simulink model "tumblingExample"  (R2020a)
settings: Solver=ode8  StartTime=0.0  StopTime=1000  FixedStep=0.1  RelTol=1e-3
values from neighbouring files (symbols this model uses):
  a = sqrt(sum(aTimesOVec.^2))    [runDocking.m]
  b = params(3)    [a_max_CLVF3D.m]    (also in forGraphingSomeBasicStuff.m = 4; runDocking.m = 15)
  finalAngle = fact*pi    (= 2.98451302091)    [runDocking.m]
  J2 = -1.08264*10^-3    (= -0.00108264)    [runDocking.m]
  ka = params(1)    [a_max_CLVF3D.m]    (also in runDocking.m = 0.01)
  kc = params(2)    [a_max_CLVF3D.m]    (also in forGraphingSomeBasicStuff.m = 1; runDocking.m = 0.01)
  kd = 5.0    (= 5)    [runDocking.m]
  MU = 3.986 * 10^5    (= 398600)    [runDocking.m]
  o_hat_B = aTimesOVec./a    [runDocking.m]
  RC_I0 = rC_I0 + RT_I0    [runDocking.m]
  RE = 6378    [runDocking.m]
  v_max = interiorPointLVF_heur(a_prime, v_max, a_max, w_max, rotNorm, dockingPortNorm, theta_d, fact, W_LVF, mu, tol, gamma, beta, muFact, muLimit)    [runDocking.m]
  VC_I0 = vC_I0 + VT_I0    [runDocking.m]
undefined symbols (not defined in the file or in its folder): A_cone, A_d, a_max, a_prime, acceptableAngle, acceptableDistance, Aeq, beq_size, C_CB, CT_BI0, d, DiscIntNeverNeededParam, FixedStep, future_time_vector, J_transverse, J_z, K, LB, m, Np, o_hat_prime, Q, RT_I0, theta_d, u_con_mat, u_con_vec, UB, VT_I0, warm_start_matrix, wT_B0, X0, x_con_mat, x_con_vec
libraries: dspsigops x1, TBMPC_Blocks x1
settings Model: Creator=hough  LastModifiedBy=hough

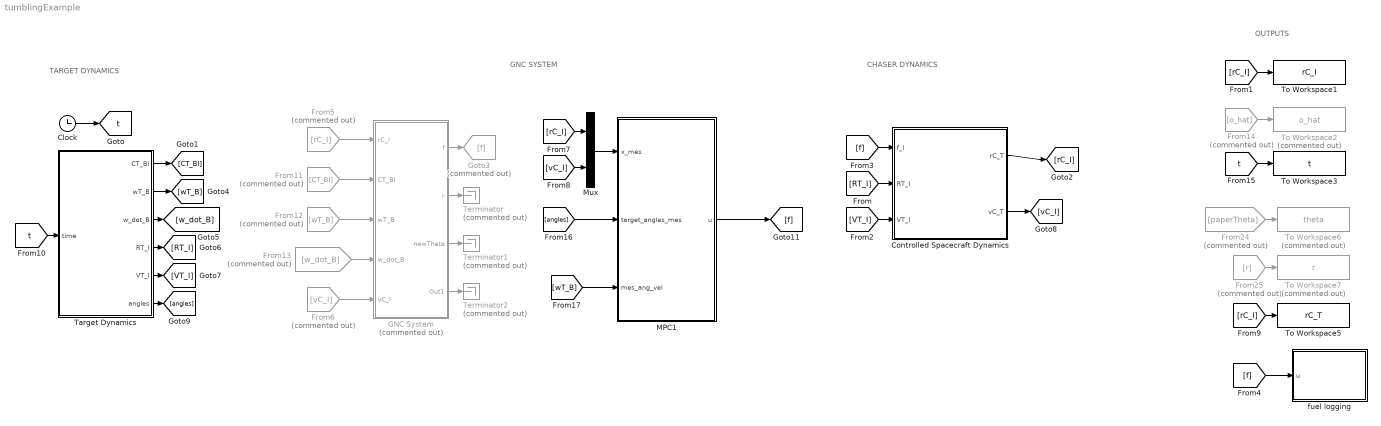
== system tumblingExample ==
  note: OUTPUTS
  note: GNC SYSTEM
  note: TARGET DYNAMICS
  note: CHASER DYNAMICS
  Clock : Clock
  Controlled Spacecraft Dynamics : Subsystem
  From11 : From  Commented=on  GotoTag=CT_BI
  From12 : From  Commented=on  GotoTag=wT_B
  From13 : From  Commented=on  GotoTag=w_dot_B
  From14 : From  Commented=on  GotoTag=o_hat
  From24 : From  Commented=on  GotoTag=paperTheta
  From25 : From  Commented=on  GotoTag=r
  From5 : From  Commented=on  GotoTag=rC_I
  From6 : From  Commented=on  GotoTag=vC_I
  GNC System : Subsystem  Commented=on
  Goto3 : Goto  Commented=on  GotoTag=f
  MPC1 : Subsystem  TreatAsAtomicUnit=on  SystemSampleTime=FixedStep  mask{t_vec=future_time_vector, J_z=J_z, J_transverse=J_transverse, u_con_mat=u_con_mat, u_con_vec=u_con_vec, x_con_mat_0=x_con_mat, x_con_vec=x_con_vec, Np=Np, d=d, A_cone=A_cone, Q=Q, Aeq=Aeq, warm_start_matrix=warm_start_matrix, A_discrete=A_d, K_feedback=K, X0=X0, beq_size=beq_size}
      mask prompts: t_vec "future time vector"; J_z "Inertia (sym axis)"; J_transverse "Inertia (trans axis)"; u_con_mat "u constraint matrix"; u_con_vec "u constraint vector"; x_con_mat_0 "x constraint matrix (proper size at least)"; x_con_vec "x constraint vector"; Np "Time horizon in steps"; d "Docking port in body-frame"; A_cone "Cone constraint matrix"; Q "Cost Matrix"; Aeq "Equality constraint matrix"; warm_start_matrix "warm start matrix"; A_discrete "A matrix (discrete system)"; K_feedback "Feedback Gain"; X0 "Initial optimizer guess"; beq_size "Height of equality matrix"
      mask help: This block runs a docking MPC controller for a axi-symmetric target spacecraft.
  Mux : Mux  Inputs=2
  Target Dynamics : Subsystem
  Terminator : Terminator  Commented=on
  Terminator1 : Terminator  Commented=on
  Terminator2 : Terminator  Commented=on
  To Workspace1 : ToWorkspace  VariableName=rC_I  SampleTime=-1
  To Workspace2 : ToWorkspace  Commented=on  VariableName=o_hat  SampleTime=-1
  To Workspace3 : ToWorkspace  VariableName=t  SampleTime=-1
  To Workspace5 : ToWorkspace  VariableName=rC_T  SampleTime=-1
  To Workspace6 : ToWorkspace  Commented=on  VariableName=theta  SampleTime=-1
  To Workspace7 : ToWorkspace  Commented=on  VariableName=r  SampleTime=-1
  fuel logging : Subsystem
  tag scope: t=global
  wires:
  GNC System/3(newTheta) -> Terminator1/1
  From12/1 -> GNC System/3(wT_B)
  From24/1 -> To Workspace6/1
  From13/1 -> GNC System/4(w_dot_B)
  From25/1 -> To Workspace7/1
  GNC System/2(r) -> Terminator/1
  [rC_I] -> To Workspace1/1
  From14/1 -> To Workspace2/1
  From11/1 -> GNC System/2(CT_BI)
  [t] -> To Workspace3/1
  Clock/1 -> [t]
  Target Dynamics/1(CT_BI) -> [CT_BI]
  Target Dynamics/2(wT_B) -> [wT_B]
  Target Dynamics/3(w_dot_B) -> [w_dot_B]
  [rC_I] -> To Workspace5/1
  Target Dynamics/4(RT_I) -> [RT_I]
  Target Dynamics/5(VT_I) -> [VT_I]
  [RT_I] -> Controlled Spacecraft Dynamics/2(RT_I)
  [VT_I] -> Controlled Spacecraft Dynamics/3(VT_I)
  GNC System/1(f) -> Goto3/1
  [f] -> Controlled Spacecraft Dynamics/1(f_I)
  [f] -> fuel logging/1(u)
  From5/1 -> GNC System/1(rC_I)
  Controlled Spacecraft Dynamics/2(vC_T) -> [vC_I]
  From6/1 -> GNC System/5(vC_I)
  [rC_I] -> Mux/1
  [vC_I] -> Mux/2
  Mux/1 -> MPC1/1(x_mes)
  GNC System/4(Out1) -> Terminator2/1
  [t] -> Target Dynamics/1(time)
  Target Dynamics/6(angles) -> [angles]
  [angles] -> MPC1/2(target_angles_mes)
  [wT_B] -> MPC1/3(mes_ang_vel)
  MPC1/1(u) -> [f]
  Controlled Spacecraft Dynamics/1(rC_T) -> [rC_I]

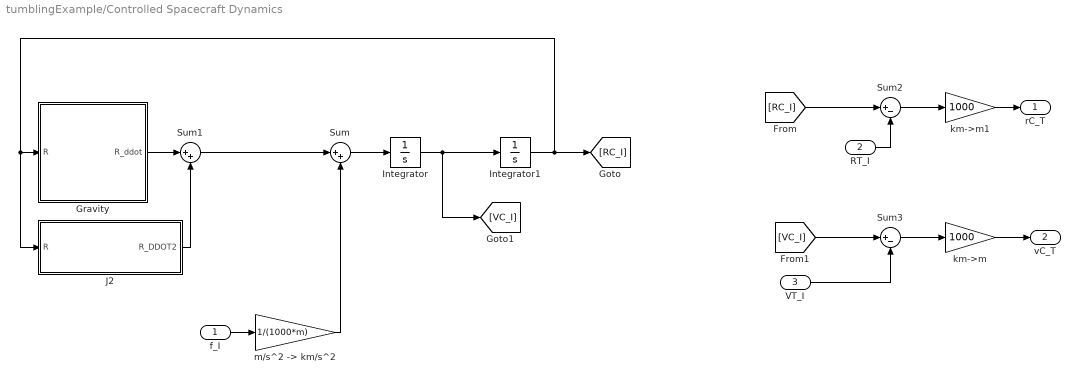
== system tumblingExample/Controlled Spacecraft Dynamics ==
  f_I : Inport
  RT_I : Inport  Port=2
  VT_I : Inport  Port=3
  Gravity : MATLAB Function  TreatAsAtomicUnit=on
  Integrator : Integrator  InitialCondition=VC_I0
  Integrator1 : Integrator  InitialCondition=RC_I0
  J2 : MATLAB Function  TreatAsAtomicUnit=on
  Sum : Sum  Inputs=|++
  Sum1 : Sum  Inputs=|++
  Sum2 : Sum  Inputs=|+-
  Sum3 : Sum  Inputs=|+-
  km->m : Gain  Gain=1000
  km->m1 : Gain  Gain=1000
  "m/s^2 -> km/s^2" : Gain  Gain=1/(1000*m)
  rC_T : Outport
  vC_T : Outport  Port=2
  wires:
  Integrator1/1 -> Gravity/1(R), J2/1(R), [RC_I]
  Integrator/1 -> Integrator1/1, [VC_I]
  Sum/1 -> Integrator/1
  f_I/1 -> "m/s^2 -> km/s^2"/1
  Gravity/1(R_ddot) -> Sum1/1
  J2/1(R_DDOT2) -> Sum1/2
  "m/s^2 -> km/s^2"/1 -> Sum/2
  Sum2/1 -> km->m1/1
  RT_I/1 -> Sum2/2
  [RC_I] -> Sum2/1
  km->m1/1 -> rC_T/1
  Sum3/1 -> km->m/1
  VT_I/1 -> Sum3/2
  [VC_I] -> Sum3/1
  km->m/1 -> vC_T/1
  Sum1/1 -> Sum/1

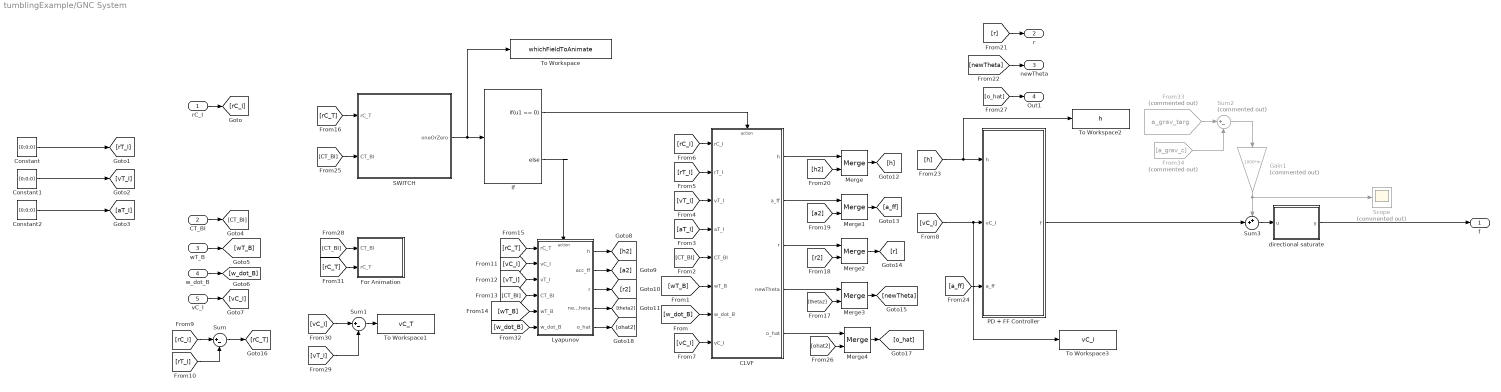
== system tumblingExample/GNC System ==
  rC_I : Inport
  CT_BI : Inport  Port=2
  wT_B : Inport  Port=3
  w_dot_B : Inport  Port=4
  vC_I : Inport  Port=5
  CLVF : Subsystem
  Constant : Constant  Value=[0;0;0]
  Constant1 : Constant  Value=[0;0;0]
  Constant2 : Constant  Value=[0;0;0]
  For Animation : Subsystem
  From33 : From  Commented=on  GotoTag=a_grav_targ  TagVisibility=global
  From34 : From  Commented=on  GotoTag=a_grav_c  TagVisibility=global
  Gain1 : Gain  Commented=on  Gain=1000*m
  If : If  IfExpression=u1 == 0
  Lyapunov : Subsystem  TreatAsAtomicUnit=on
  Merge{,1..4} (5 alike) : Merge
  PD + FF Controller : MATLAB Function  TreatAsAtomicUnit=on
  SWITCH : Subsystem
  Scope : Scope  Commented=on
  Sum : Sum  Inputs=|+-
  Sum1 : Sum  Inputs=|+-
  Sum2 : Sum  Commented=on  Inputs=|+-
  Sum3 : Sum  Inputs=++|
  To Workspace : ToWorkspace  VariableName=whichFieldToAnimate  SampleTime=-1
  To Workspace1 : ToWorkspace  VariableName=vC_T  SampleTime=-1
  To Workspace2 : ToWorkspace  VariableName=h  SampleTime=-1
  To Workspace3 : ToWorkspace  VariableName=vC_I  SampleTime=-1
  directional saturate : MATLAB Function  TreatAsAtomicUnit=on
  f : Outport
  r : Outport  Port=2
  newTheta : Outport  Port=3
  Out1 : Outport  Port=4
  wires:
  rC_I/1 -> [rC_I]
  CT_BI/1 -> [CT_BI]
  wT_B/1 -> [wT_B]
  w_dot_B/1 -> [w_dot_B]
  vC_I/1 -> [vC_I]
  [vC_I] -> To Workspace3/1, PD + FF Controller/2(vC_I)
  [rC_I] -> CLVF/1(rC_I)
  [rT_I] -> CLVF/2(rT_I)
  [vT_I] -> CLVF/3(vT_I)
  [aT_I] -> CLVF/4(aT_I)
  [CT_BI] -> CLVF/5(CT_BI)
  [wT_B] -> CLVF/6(wT_B)
  [w_dot_B] -> CLVF/7(w_dot_B)
  [vC_I] -> CLVF/8(vC_I)
  If/1 -> CLVF/Action
  CLVF/1(h) -> Merge/1
  CLVF/2(a_ff) -> Merge1/1
  CLVF/3(r) -> Merge2/1
  CLVF/4(newTheta) -> Merge3/1
  [theta2] -> Merge3/2
  [r2] -> Merge2/2
  [a2] -> Merge1/2
  [h2] -> Merge/2
  Merge/1 -> [h]
  Merge1/1 -> [a_ff]
  Merge2/1 -> [r]
  Merge3/1 -> [newTheta]
  [r] -> r/1
  [newTheta] -> newTheta/1
  [h] -> To Workspace2/1, PD + FF Controller/1(h)
  [a_ff] -> PD + FF Controller/3(a_ff)
  If/2 -> Lyapunov/Action
  [rC_I] -> Sum/1
  [rT_I] -> Sum/2
  Lyapunov/1(h) -> [h2]
  Lyapunov/2(acc_ff) -> [a2]
  Lyapunov/3(r) -> [r2]
  Lyapunov/4(newTheta) -> [theta2]
  [vC_I] -> Lyapunov/2(vC_I)
  [vT_I] -> Lyapunov/3(vT_I)
  SWITCH/1(oneOrZero) -> To Workspace/1, If/1
  Sum/1 -> [rC_T]
  [rC_T] -> Lyapunov/1(rC_T)
  [rC_T] -> SWITCH/1(rC_T)
  Merge4/1 -> [o_hat]
  CLVF/5(o_hat) -> Merge4/1
  [ohat2] -> Merge4/2
  Lyapunov/5(o_hat) -> [ohat2]
  [o_hat] -> Out1/1
  [vC_I] -> Sum1/1
  [vT_I] -> Sum1/2
  Sum1/1 -> To Workspace1/1
  [rC_T] -> For Animation/2(rC_T)
  [CT_BI] -> Lyapunov/4(CT_BI)
  [wT_B] -> Lyapunov/5(wT_B)
  [w_dot_B] -> Lyapunov/6(w_dot_B)
  [CT_BI] -> SWITCH/2(CT_BI)
  [CT_BI] -> For Animation/1(CT_BI)
  PD + FF Controller/1(f) -> Sum3/2
  directional saturate/1(y) -> f/1
  Sum2/1 -> Gain1/1
  From34/1 -> Sum2/2
  From33/1 -> Sum2/1
  Gain1/1 -> Sum3/1, Scope/1
  Sum3/1 -> directional saturate/1(u)
  Constant/1 -> [rT_I]
  Constant1/1 -> [vT_I]
  Constant2/1 -> [aT_I]

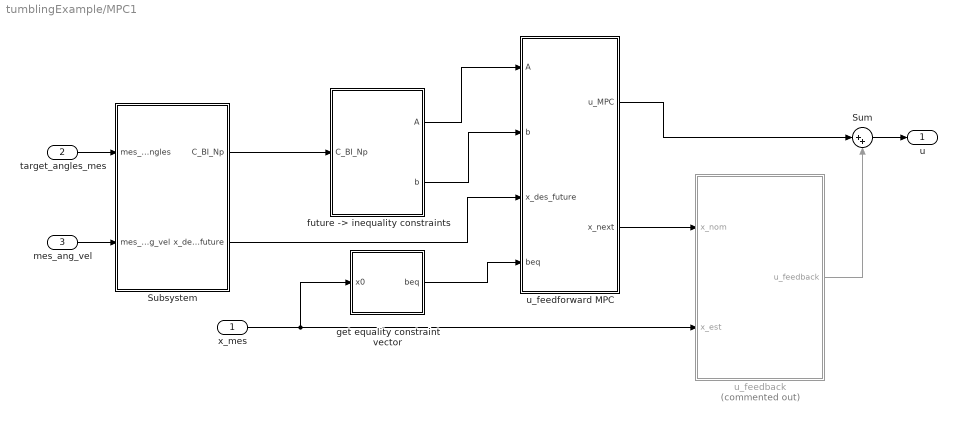
== system tumblingExample/MPC1 ==
  x_mes : Inport
  target_angles_mes : Inport  Port=2
  mes_ang_vel : Inport  Port=3
  Subsystem : Subsystem
  Sum : Sum  Inputs=|++
  "future -> inequality constraints" : Subsystem
  get equality constraint vector : Subsystem
  u_feedback : Subsystem  Commented=on
  u_feedforward MPC : Subsystem
  u : Outport
  wires:
  u_feedforward MPC/1(u_MPC) -> Sum/1
  Sum/1 -> u/1
  x_mes/1 -> get equality constraint vector/1(x0), u_feedback/2(x_est)
  u_feedforward MPC/2(x_next) -> u_feedback/1(x_nom)
  u_feedback/1(u_feedback) -> Sum/2
  "future -> inequality constraints"/1(A) -> u_feedforward MPC/1(A)
  "future -> inequality constraints"/2(b) -> u_feedforward MPC/2(b)
  Subsystem/1(C_BI_Np) -> "future -> inequality constraints"/1(C_BI_Np)
  target_angles_mes/1 -> Subsystem/1(mes_angles)
  mes_ang_vel/1 -> Subsystem/2(mes_ang_vel)
  Subsystem/2(x_des_future) -> u_feedforward MPC/3(x_des_future)
  get equality constraint vector/1(beq) -> u_feedforward MPC/4(beq)

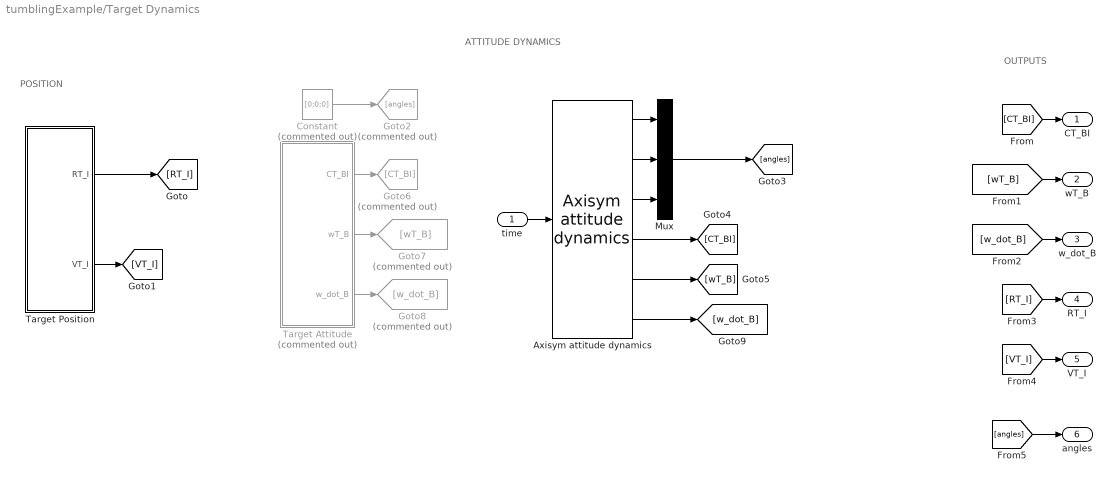
== system tumblingExample/Target Dynamics ==
  note: POSITION
  note: ATTITUDE DYNAMICS
  note: OUTPUTS
  time : Inport
  Axisym attitude dynamics : TBMPC_Blocks/Axisym attitude dynamics  J_transverse=J_transverse  J_z=J_z  omega_t=w_t  omega_z=w_z  mu_0=mu0  gamma_0=gamma  theta_0=theta0
  Constant : Constant  Commented=on  Value=[0;0;0]
  Goto2 : Goto  Commented=on  GotoTag=angles
  Goto6 : Goto  Commented=on  GotoTag=CT_BI
  Goto7 : Goto  Commented=on  GotoTag=wT_B
  Goto8 : Goto  Commented=on  GotoTag=w_dot_B
  Mux : Mux  Inputs=3
  Target Attitude : Subsystem  Commented=on
  Target Position : Subsystem
  CT_BI : Outport
  wT_B : Outport  Port=2
  w_dot_B : Outport  Port=3
  RT_I : Outport  Port=4
  VT_I : Outport  Port=5
  angles : Outport  Port=6
  wires:
  Target Attitude/3(w_dot_B) -> Goto8/1
  Target Attitude/1(CT_BI) -> Goto6/1
  Target Attitude/2(wT_B) -> Goto7/1
  [CT_BI] -> CT_BI/1
  [wT_B] -> wT_B/1
  [w_dot_B] -> w_dot_B/1
  Target Position/2(VT_I) -> [VT_I]
  [RT_I] -> RT_I/1
  [VT_I] -> VT_I/1
  time/1 -> Axisym attitude dynamics/1
  Axisym attitude dynamics/1 -> Mux/1
  Axisym attitude dynamics/2 -> Mux/2
  Axisym attitude dynamics/3 -> Mux/3
  [angles] -> angles/1
  Constant/1 -> Goto2/1
  Mux/1 -> [angles]
  Axisym attitude dynamics/4 -> [CT_BI]
  Axisym attitude dynamics/5 -> [wT_B]
  Axisym attitude dynamics/6 -> [w_dot_B]
  Target Position/1(RT_I) -> [RT_I]

== system tumblingExample/fuel logging ==
  u : Inport
  F->acc : Gain  Gain=1/m
  Gain : Gain  Gain=1/m
  To Workspace4 : ToWorkspace  VariableName=a_norm  SampleTime=-1
  To Workspace8 : ToWorkspace  VariableName=F_act  SampleTime=-1
  acc->delV : DiscreteIntegrator  SampleTime=-1  ICPrevOutput=DiscIntNeverNeededParam  ICPrevScaledInput=DiscIntNeverNeededParam
  get Norm : MATLAB Function  TreatAsAtomicUnit=on
  getNorm : MATLAB Function  TreatAsAtomicUnit=on
  wires:
  getNorm/1(y) -> Gain/1
  get Norm/1(y) -> acc->delV/1
  acc->delV/1 -> To Workspace8/1
  F->acc/1 -> get Norm/1(u)
  Gain/1 -> To Workspace4/1
  u/1 -> F->acc/1, getNorm/1(u)

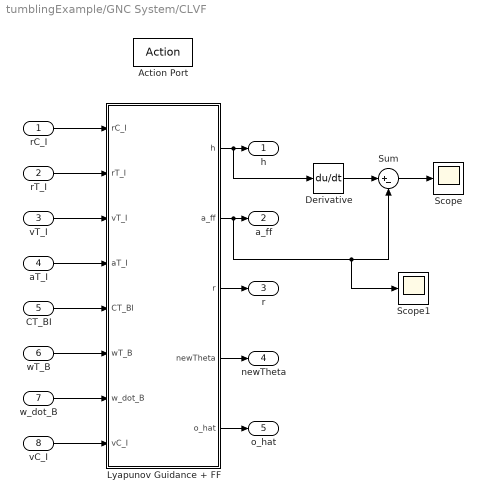
== system tumblingExample/GNC System/CLVF ==
  rC_I : Inport
  rT_I : Inport  Port=2
  vT_I : Inport  Port=3
  aT_I : Inport  Port=4
  CT_BI : Inport  Port=5
  wT_B : Inport  Port=6
  w_dot_B : Inport  Port=7
  vC_I : Inport  Port=8
  Action Port : ActionPort  ActionPortLabel=if(u1 == 0)
  Derivative : Derivative
  Lyapunov Guidance + FF : MATLAB Function  TreatAsAtomicUnit=on
  Scope : Scope
  Scope1 : Scope
  Sum : Sum  Inputs=|+-
  h : Outport
  a_ff : Outport  Port=2
  r : Outport  Port=3
  newTheta : Outport  Port=4
  o_hat : Outport  Port=5
  wires:
  vT_I/1 -> Lyapunov Guidance + FF/3(vT_I)
  rT_I/1 -> Lyapunov Guidance + FF/2(rT_I)
  wT_B/1 -> Lyapunov Guidance + FF/6(wT_B)
  w_dot_B/1 -> Lyapunov Guidance + FF/7(w_dot_B)
  vC_I/1 -> Lyapunov Guidance + FF/8(vC_I)
  CT_BI/1 -> Lyapunov Guidance + FF/5(CT_BI)
  aT_I/1 -> Lyapunov Guidance + FF/4(aT_I)
  rC_I/1 -> Lyapunov Guidance + FF/1(rC_I)
  Lyapunov Guidance + FF/3(r) -> r/1
  Lyapunov Guidance + FF/2(a_ff) -> Scope1/1, Sum/2, a_ff/1
  Lyapunov Guidance + FF/1(h) -> Derivative/1, h/1
  Lyapunov Guidance + FF/4(newTheta) -> newTheta/1
  Lyapunov Guidance + FF/5(o_hat) -> o_hat/1
  Derivative/1 -> Sum/1
  Sum/1 -> Scope/1

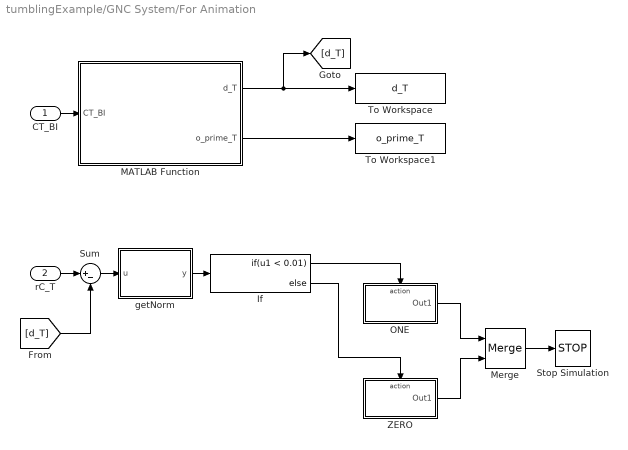
== system tumblingExample/GNC System/For Animation ==
  CT_BI : Inport
  rC_T : Inport  Port=2
  If : If  IfExpression=u1 < 0.01
  MATLAB Function : MATLAB Function  TreatAsAtomicUnit=on
  Merge : Merge
  ONE : Subsystem  TreatAsAtomicUnit=on
  Stop Simulation : Stop
  Sum : Sum  Inputs=|+-
  To Workspace : ToWorkspace  VariableName=d_T  SampleTime=-1
  To Workspace1 : ToWorkspace  VariableName=o_prime_T  SampleTime=-1
  ZERO : Subsystem  TreatAsAtomicUnit=on
  getNorm : MATLAB Function  TreatAsAtomicUnit=on
  wires:
  CT_BI/1 -> MATLAB Function/1(CT_BI)
  MATLAB Function/1(d_T) -> [d_T], To Workspace/1
  MATLAB Function/2(o_prime_T) -> To Workspace1/1
  rC_T/1 -> Sum/1
  [d_T] -> Sum/2
  Sum/1 -> getNorm/1(u)
  getNorm/1(y) -> If/1
  If/1 -> ONE/Action
  If/2 -> ZERO/Action
  ONE/1(Out1) -> Merge/1
  ZERO/1(Out1) -> Merge/2
  Merge/1 -> Stop Simulation/1

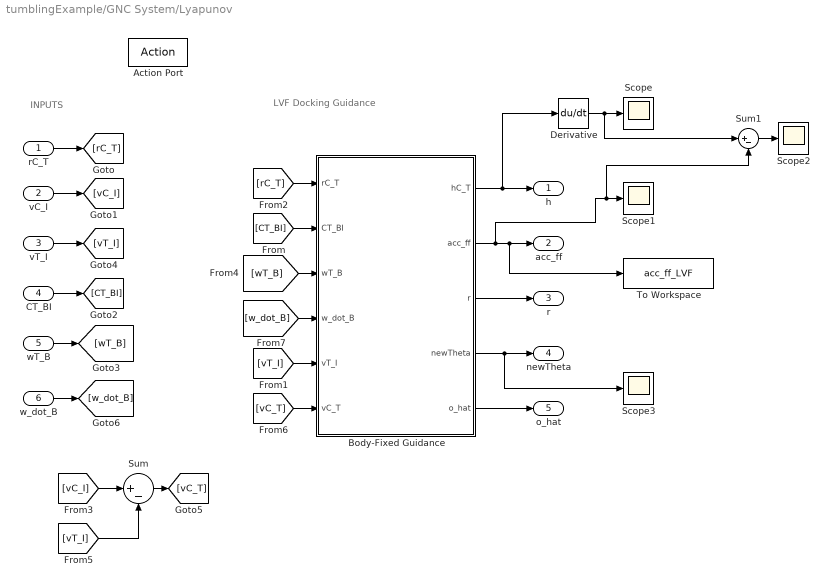
== system tumblingExample/GNC System/Lyapunov ==
  note: LVF Docking Guidance
  note: INPUTS
  rC_T : Inport
  vC_I : Inport  Port=2
  vT_I : Inport  Port=3
  CT_BI : Inport  Port=4
  wT_B : Inport  Port=5
  w_dot_B : Inport  Port=6
  Action Port : ActionPort  ActionPortLabel=else
  Body-Fixed Guidance : MATLAB Function  TreatAsAtomicUnit=on
  Derivative : Derivative
  Scope{,1..3} (4 alike) : Scope
  Sum : Sum  Inputs=|+-
  Sum1 : Sum  Inputs=|+-
  To Workspace : ToWorkspace  VariableName=acc_ff_LVF  SampleTime=-1
  h : Outport
  acc_ff : Outport  Port=2
  r : Outport  Port=3
  newTheta : Outport  Port=4
  o_hat : Outport  Port=5
  wires:
  rC_T/1 -> [rC_T]
  vC_I/1 -> [vC_I]
  CT_BI/1 -> [CT_BI]
  wT_B/1 -> [wT_B]
  [rC_T] -> Body-Fixed Guidance/1(rC_T)
  [wT_B] -> Body-Fixed Guidance/3(wT_B)
  [CT_BI] -> Body-Fixed Guidance/2(CT_BI)
  [w_dot_B] -> Body-Fixed Guidance/4(w_dot_B)
  vT_I/1 -> [vT_I]
  Body-Fixed Guidance/1(hC_T) -> Derivative/1, h/1
  [vT_I] -> Body-Fixed Guidance/5(vT_I)
  Body-Fixed Guidance/3(r) -> r/1
  Body-Fixed Guidance/4(newTheta) -> Scope3/1, newTheta/1
  Body-Fixed Guidance/5(o_hat) -> o_hat/1
  [vC_I] -> Sum/1
  [vT_I] -> Sum/2
  Sum/1 -> [vC_T]
  [vC_T] -> Body-Fixed Guidance/6(vC_T)
  Body-Fixed Guidance/2(acc_ff) -> To Workspace/1, acc_ff/1, Sum1/2, Scope1/1
  Derivative/1 -> Sum1/1, Scope/1
  Sum1/1 -> Scope2/1
  w_dot_B/1 -> [w_dot_B]

== system tumblingExample/GNC System/SWITCH ==
  rC_T : Inport
  CT_BI : Inport  Port=2
  Delay : Delay  DelayLength=1  InitialCondition=0
  Sample and Hold : dspsigops/Sample and Hold  trig=Rising edge  initCond=0  latchinput=off
  inDesiredRadius : MATLAB Function  TreatAsAtomicUnit=on
  sufficientTime : MATLAB Function  TreatAsAtomicUnit=on
  oneOrZero : Outport
  wires:
  rC_T/1 -> inDesiredRadius/1(rC_T)
  CT_BI/1 -> inDesiredRadius/2(CT_BI)
  Delay/1 -> inDesiredRadius/3(currentCnt)
  inDesiredRadius/1(newCnt) -> sufficientTime/1(cnt), Delay/1
  Sample and Hold/1 -> oneOrZero/1
  sufficientTime/1(oneOrZero) -> Sample and Hold/Trigger, Sample and Hold/1

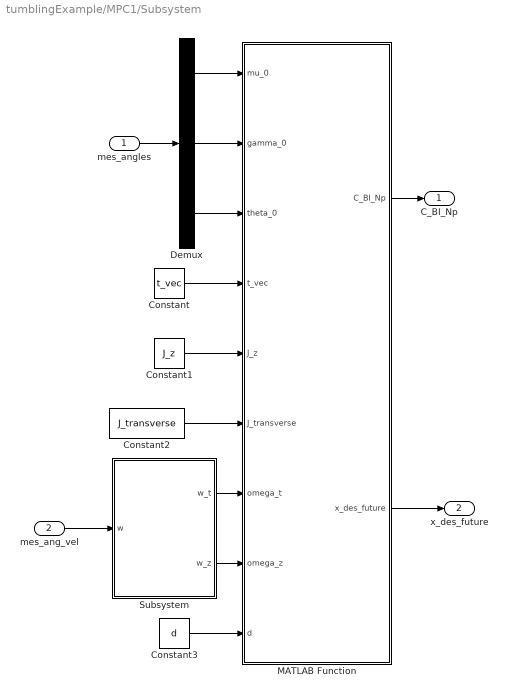
== system tumblingExample/MPC1/Subsystem ==
  mes_angles : Inport
  mes_ang_vel : Inport  Port=2
  Constant : Constant  Value=t_vec
  Constant1 : Constant  Value=J_z
  Constant2 : Constant  Value=J_transverse
  Constant3 : Constant  Value=d
  Demux : Demux  Outputs=3
  MATLAB Function : MATLAB Function  TreatAsAtomicUnit=on
  Subsystem : Subsystem
  C_BI_Np : Outport
  x_des_future : Outport  Port=2
  wires:
  MATLAB Function/1(C_BI_Np) -> C_BI_Np/1
  MATLAB Function/2(x_des_future) -> x_des_future/1
  Constant/1 -> MATLAB Function/4(t_vec)
  Demux/2 -> MATLAB Function/2(gamma_0)
  Demux/3 -> MATLAB Function/3(theta_0)
  Demux/1 -> MATLAB Function/1(mu_0)
  mes_angles/1 -> Demux/1
  Constant2/1 -> MATLAB Function/6(J_transverse)
  Constant1/1 -> MATLAB Function/5(J_z)
  mes_ang_vel/1 -> Subsystem/1(w)
  Subsystem/1(w_t) -> MATLAB Function/7(omega_t)
  Subsystem/2(w_z) -> MATLAB Function/8(omega_z)
  Constant3/1 -> MATLAB Function/9(d)

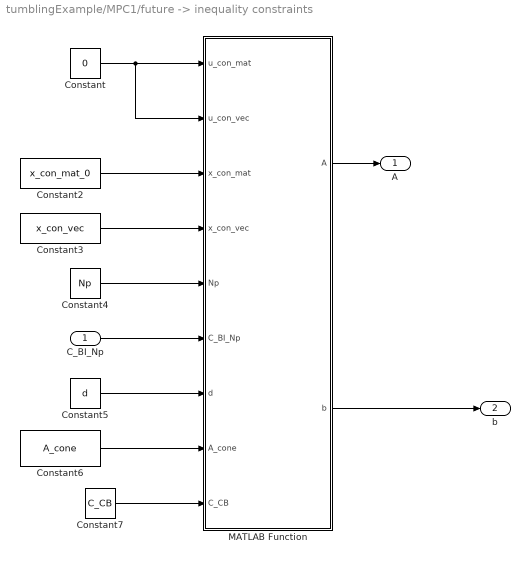
== system tumblingExample/MPC1/future -> inequality constraints ==
  C_BI_Np : Inport
  Constant : Constant  Value=0
  Constant2 : Constant  Value=x_con_mat_0
  Constant3 : Constant  Value=x_con_vec
  Constant4 : Constant  Value=Np
  Constant5 : Constant  Value=d
  Constant6 : Constant  Value=A_cone
  Constant7 : Constant  Value=C_CB
  MATLAB Function : MATLAB Function  TreatAsAtomicUnit=on
  A : Outport
  b : Outport  Port=2
  wires:
  MATLAB Function/1(A) -> A/1
  C_BI_Np/1 -> MATLAB Function/6(C_BI_Np)
  Constant2/1 -> MATLAB Function/3(x_con_mat)
  Constant3/1 -> MATLAB Function/4(x_con_vec)
  Constant4/1 -> MATLAB Function/5(Np)
  Constant5/1 -> MATLAB Function/7(d)
  Constant6/1 -> MATLAB Function/8(A_cone)
  Constant7/1 -> MATLAB Function/9(C_CB)
  MATLAB Function/2(b) -> b/1
  Constant/1 -> MATLAB Function/2(u_con_vec), MATLAB Function/1(u_con_mat)

== system tumblingExample/MPC1/get equality constraint vector ==
  x0 : Inport
  Constant : Constant  Value=Np
  Constant1 : Constant  Value=A_discrete
  Gain : Gain  Gain=-1
  MATLAB Function : MATLAB Function  TreatAsAtomicUnit=on
  beq : Outport
  wires:
  x0/1 -> MATLAB Function/3(x0)
  Constant/1 -> MATLAB Function/2(Np)
  Constant1/1 -> MATLAB Function/1(A)
  Gain/1 -> beq/1
  MATLAB Function/1(p) -> Gain/1

== system tumblingExample/MPC1/u_feedback ==
  x_nom : Inport
  x_est : Inport  Port=2
  Constant : Constant  Value=K_feedback
  Matrix Multiply : Product  Multiplication=Matrix(*)
  Sum : Sum  Inputs=|+-
  u_feedback : Outport
  wires:
  x_nom/1 -> Sum/1
  x_est/1 -> Sum/2
  Sum/1 -> Matrix Multiply/2
  Constant/1 -> Matrix Multiply/1
  Matrix Multiply/1 -> u_feedback/1

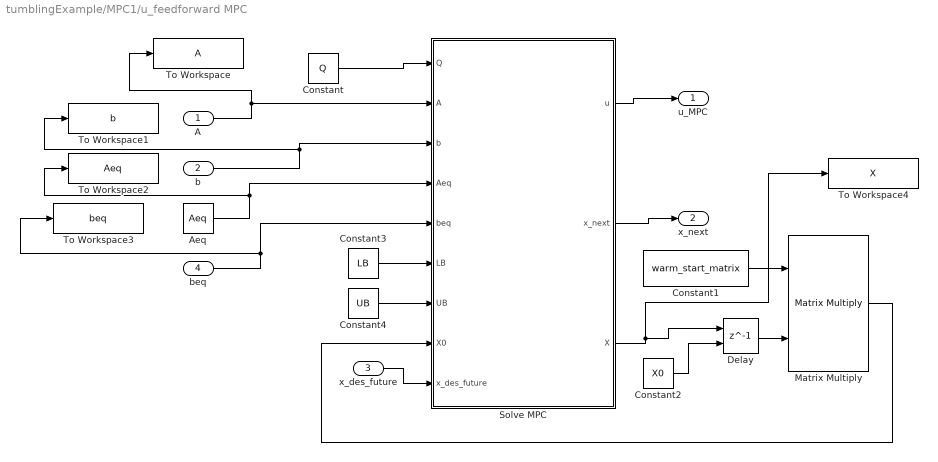
== system tumblingExample/MPC1/u_feedforward MPC ==
  A : Inport
  b : Inport  Port=2
  x_des_future : Inport  Port=3
  beq : Inport  Port=4
  Aeq : Constant  Value=Aeq
  Constant : Constant  Value=Q
  Constant1 : Constant  Value=warm_start_matrix
  Constant2 : Constant  Value=X0
  Constant3 : Constant  Value=LB
  Constant4 : Constant  Value=UB
  Delay : Delay  DelayLength=1  InitialConditionSource=Input port
      settings: InputPortMap=u0,p4
  Matrix Multiply : Product  Multiplication=Matrix(*)
  Solve MPC : MATLAB Function  TreatAsAtomicUnit=on
  To Workspace : ToWorkspace  VariableName=A  SaveFormat=Structure  SampleTime=-1
  To Workspace1 : ToWorkspace  VariableName=b  SaveFormat=Structure  SampleTime=-1
  To Workspace2 : ToWorkspace  VariableName=Aeq  SampleTime=-1
  To Workspace3 : ToWorkspace  VariableName=beq  SaveFormat=Structure  SampleTime=-1
  To Workspace4 : ToWorkspace  VariableName=X  SampleTime=-1
  u_MPC : Outport
  x_next : Outport  Port=2
  wires:
  A/1 -> To Workspace/1, Solve MPC/2(A)
  Matrix Multiply/1 -> Solve MPC/8(X0)
  beq/1 -> To Workspace3/1, Solve MPC/5(beq)
  Constant1/1 -> Matrix Multiply/1
  Constant/1 -> Solve MPC/1(Q)
  Delay/1 -> Matrix Multiply/2
  Aeq/1 -> To Workspace2/1, Solve MPC/4(Aeq)
  b/1 -> To Workspace1/1, Solve MPC/3(b)
  Solve MPC/3(X) -> To Workspace4/1, Delay/1
  Solve MPC/1(u) -> u_MPC/1
  Solve MPC/2(x_next) -> x_next/1
  x_des_future/1 -> Solve MPC/9(x_des_future)
  Constant2/1 -> Delay/2
  Constant3/1 -> Solve MPC/6(LB)
  Constant4/1 -> Solve MPC/7(UB)

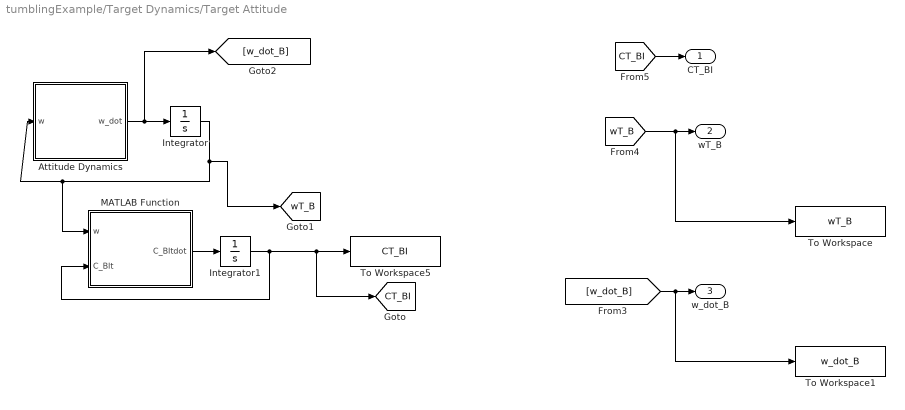
== system tumblingExample/Target Dynamics/Target Attitude ==
  Attitude Dynamics : MATLAB Function  TreatAsAtomicUnit=on
  Integrator : Integrator  InitialCondition=wT_B0
  Integrator1 : Integrator  InitialCondition=CT_BI0
  MATLAB Function : MATLAB Function  TreatAsAtomicUnit=on
  To Workspace : ToWorkspace  VariableName=wT_B  SampleTime=-1
  To Workspace1 : ToWorkspace  VariableName=w_dot_B  SampleTime=-1
  To Workspace5 : ToWorkspace  VariableName=CT_BI  SampleTime=-1
  CT_BI : Outport
  wT_B : Outport  Port=2
  w_dot_B : Outport  Port=3
  tag scope: CT_BI=global, wT_B=global
  wires:
  [CT_BI] -> CT_BI/1
  [wT_B] -> To Workspace/1, wT_B/1
  [w_dot_B] -> To Workspace1/1, w_dot_B/1
  MATLAB Function/1(C_BItdot) -> Integrator1/1
  Integrator1/1 -> MATLAB Function/2(C_BIt), [CT_BI], To Workspace5/1
  Integrator/1 -> [wT_B], MATLAB Function/1(w), Attitude Dynamics/1(w)
  Attitude Dynamics/1(w_dot) -> [w_dot_B], Integrator/1

== system tumblingExample/Target Dynamics/Target Position ==
  Gravity : MATLAB Function  TreatAsAtomicUnit=on
  Integrator : Integrator  InitialCondition=VT_I0
  Integrator1 : Integrator  InitialCondition=RT_I0
  J2 : MATLAB Function  TreatAsAtomicUnit=on
  Sum : Sum  Inputs=|++
  RT_I : Outport
  VT_I : Outport  Port=2
  tag scope: a_grav_targ=global
  wires:
  Integrator/1 -> VT_I/1, Integrator1/1
  Integrator1/1 -> RT_I/1, J2/1(R), Gravity/1(R)
  Gravity/1(R_ddot) -> Sum/1
  J2/1(R_DDOT2) -> Sum/2
  Sum/1 -> [a_grav_targ], Integrator/1

== system tumblingExample/GNC System/For Animation/ONE ==
  Action Port : ActionPort  ActionPortLabel=if(u1 < 0.01)
  Constant : Constant
  Out1 : Outport
  wires:
  Constant/1 -> Out1/1

== system tumblingExample/GNC System/For Animation/ZERO ==
  Action Port : ActionPort  ActionPortLabel=else
  Constant : Constant  Value=0
  Out1 : Outport
  wires:
  Constant/1 -> Out1/1

== system tumblingExample/MPC1/Subsystem/Subsystem ==
  w : Inport
  Add : Sum
  Demux1 : Demux  Outputs=3
  Sqrt : Sqrt  SaturateOnIntegerOverflow=on
  Square : Math  Operator=square  SaturateOnIntegerOverflow=on
  Square1 : Math  Operator=square  SaturateOnIntegerOverflow=on
  w_t : Outport
  w_z : Outport  Port=2
  wires:
  Square/1 -> Add/1
  Demux1/1 -> Square/1
  Demux1/2 -> Square1/1
  Add/1 -> Sqrt/1
  Square1/1 -> Add/2
  w/1 -> Demux1/1
  Demux1/3 -> w_z/1
  Sqrt/1 -> w_t/1

== matlab function tumblingExample/MPC1/Subsystem/MATLAB Function ==
  data: mu_0 input; C_BI_Np output; gamma_0 input; theta_0 input; t_vec input; J_z input; J_transverse input; omega_t input; omega_z input; x_des_future output; d input
function [C_BI_Np, x_des_future] = fcn(mu_0, gamma_0, theta_0, t_vec, J_z, J_transverse, omega_t, omega_z, d)

    [C_BI_Np, x_des_future] = return_C_BI_from_axisym(mu_0, gamma_0, theta_0, t_vec, J_z, J_transverse, omega_z, omega_t, d);


end

== matlab function tumblingExample/Target Dynamics/Target Attitude/MATLAB Function ==
  data: w input; C_BItdot output; C_BIt input
function C_BItdot = fcn(w,C_BIt)

w_skew = [0 -w(3) w(2)
          w(3) 0 -w(1)
          -w(2) w(1) 0];

C_BItdot = -w_skew*C_BIt;

== matlab function tumblingExample/GNC System/SWITCH/sufficientTime ==
  data: oneOrZero output; cnt input; cntThreshold parameter
function oneOrZero = fcn(cnt, cntThreshold)

    if cnt < cntThreshold
        oneOrZero = 0; % Not enough.
    else
        oneOrZero = 1;
    end
end

== matlab function tumblingExample/fuel logging/getNorm ==
  data: u input; y output
function y = fcn(u)

y = sqrt(sum(u.^2));

== matlab function tumblingExample/Controlled Spacecraft Dynamics/J2 ==
  data: R input; R_DDOT2 output; MU parameter; J2 parameter; RE parameter
function R_DDOT2 = fcn(R, MU, J2, RE)

R_norm = sqrt(sum(R.^2));

R_DDOT2_part1 = 3*MU*J2*RE^2/(2*R_norm^5);

R_DDOT2_part2 = (  5*(R(3))^2/R_norm^2  -  1  )*R;

R_DDOT2_part3 =  -2*R(3)*[0;0;1];

R_DDOT2 = R_DDOT2_part1  *  (R_DDOT2_part2 + R_DDOT2_part3);

== matlab function tumblingExample/GNC System/For Animation/MATLAB Function ==
  data: CT_BI input; d_T output; d parameter; o_prime_T output; o_hat_prime parameter
function [d_T, o_prime_T] = fcn(CT_BI,d, o_hat_prime)
    
    C_IB = CT_BI';
    d_T = C_IB*d;
    o_prime_T = C_IB*o_hat_prime;
    
end

== matlab function tumblingExample/MPC1/future -> inequality constraints/MATLAB Function ==
  data: u_con_mat input; A output size=A_size; u_con_vec input; x_con_mat input; x_con_vec input; Np input; C_BI_Np input; d input; A_cone input; b output size=b_size; C_CB input
function [A, b] = fcn(u_con_mat, u_con_vec, x_con_mat, x_con_vec, Np, C_BI_Np, d, A_cone, C_CB)

% Note, u_con_mat and u_con_vec are left here in case I want to put them
% back in...

    [A, b] = return_inequality_con_mat_and_vec(x_con_mat, x_con_vec, Np, [], [], C_BI_Np, d, A_cone, C_CB);

end

== matlab function tumblingExample/GNC System/Lyapunov/Body-Fixed Guidance ==
  data: rC_T input; hC_T output; CT_BI input; wT_B input; v_max parameter; d parameter; o_hat_prime parameter; theta_d parameter; a_prime parameter; acc_ff output; w_dot_B input; r output; newTheta output; vT_I input; o_hat output; finalAngle parameter; vC_T input
function [hC_T, acc_ff, r, newTheta, o_hat] = lyapVecField(rC_T, CT_BI, wT_B, v_max, d, o_hat_prime, theta_d, a_prime, w_dot_B, vT_I, finalAngle, vC_T)

%     C_BIt = C3(theta);
    C_IB = CT_BI';
    
%     w_OI = [0;0;theta_dot];
%     w_dot_OI = [0;0;theta_ddot];

    wT_I = C_IB*wT_B;
    w_dot_I = C_IB*w_dot_B;
    
    o_hat_B = o_hat_prime;
    
    o_hat = C_IB * o_hat_prime;
    
    % The velocity of the "target" is actually the velocity of the docking
    % port!
        vD_I = vT_I + skew(wT_I)*(C_IB * d);
        vC_D = vC_T - (C_IB* skew(wT_B)* d);
        
    % The position relative to the target is actaully the position relative
    % to the docking port:
        rD_T = C_IB*d;
        rC_D = rC_T - rD_T;
        
%         rC_D_B = CT_BI*rC_T - d;
%         r_mag = sqrt(sum(rC_D_B.^2));
%         
%     % Get some other theta:
%         someothertheta = acos(o_hat_prime'*rC_D_B/(r_mag*sqrt(sum(o_hat_prime.^2)));
        
    % The acceleration of the target is just the acceleration of the
    % docking port:
        aD_I = C_IB*(skew(wT_B)*skew(wT_B)*d + skew(w_dot_B)*d) ; % Assuming that omega_dot == 0.
    
    % w_dot = [0;0;theta_ddot]; Will be needed for the acc_ff
    
        q = 0.0001; % Small number!
% q = 0;

    [hC_T, acc_ff, r, newTheta] = LVF(rC_D, o_hat, q, v_max, theta_d, wT_I, vD_I, a_prime, finalAngle, vC_D, aD_I, w_dot_I, d, o_hat_B, CT_BI);
    
end

== matlab function tumblingExample/MPC1/get equality constraint vector/MATLAB Function ==
  data: A input; p output size=beq_size; Np input; x0 input
function p = fcn(A, Np, x0)
    p = return_equality_vec(A, Np, x0);

end

== matlab function tumblingExample/GNC System/For Animation/getNorm ==
  data: u input; y output
function y = fcn(u)

y = sqrt(sum(u.^2));

== matlab function tumblingExample/Target Dynamics/Target Position/Gravity ==
  data: R input; R_ddot output; MU parameter
function R_ddot = fcn(R, MU)

r_norm = sqrt(sum(R.^2));
R_ddot = -MU/r_norm^3  *  R;

== matlab function tumblingExample/Target Dynamics/Target Position/J2 ==
  data: R input; R_DDOT2 output; MU parameter; J2 parameter; RE parameter
function R_DDOT2 = fcn(R, MU, J2, RE)

R_norm = sqrt(sum(R.^2));

R_DDOT2_part1 = 3*MU*J2*RE^2/(2*R_norm^5);

R_DDOT2_part2 = (  5*(R(3))^2/R_norm^2  -  1  )*R;

R_DDOT2_part3 =  -2*R(3)*[0;0;1];

R_DDOT2 = R_DDOT2_part1  *  (R_DDOT2_part2 + R_DDOT2_part3);

== matlab function tumblingExample/fuel logging/get Norm ==
  data: u input; y output
function y = fcn(u)

y = sqrt(sum(u.^2));

== matlab function tumblingExample/GNC System/directional saturate ==
  data: u input; y output; a_max parameter; m parameter
function y = fcn(u, a_max, m)

    u_max = a_max*m;
    
    if sqrt(sum(u.^2)) <= u_max
        y = u;
    else
        y = u./sqrt(sum(u.^2)) * u_max;
    end

== matlab function tumblingExample/MPC1/u_feedforward MPC/Solve MPC ==
  data: Q input; u output; x_next output; A input size=A_size; b input size=b_size; Aeq input; beq input size=beq_size; LB input; UB input; X0 input; X output; x_des_future input
function [u, x_next, X] = MPC(Q, A, b, Aeq, beq, LB, UB, X0, x_des_future)

    % solve the full time-horizon (states + inputs) (should probably set
    % this outside of simulink...)
    options = optimoptions('quadprog', 'Algorithm','active-set', 'Display','off');
    linear_vec = (-2*Q'*x_des_future);
    X = quadprog(2*Q, linear_vec, A, b, Aeq, beq, LB, UB, X0, options);

    % get the input only (first timestep)
    u = zeros(3,1);
    u(:) = X(1:3);
    
    % get the next desired state (3 for vel, 3 for pos)
    x_next = zeros(6,1);
    x_next(:) = X(4:9);
    
end

== matlab function tumblingExample/GNC System/SWITCH/inDesiredRadius ==
  data: rC_T input; newCnt output; CT_BI input; currentCnt input; o_hat_B parameter; a parameter; acceptableAngle parameter; acceptableDistance parameter
function newCnt = accumulateTimeInRadius(rC_T, CT_BI, currentCnt, o_hat_B, a, acceptableAngle, acceptableDistance)

% Check whether we are in the acceptable radius
        C_IB = CT_BI';
%         desiredPosition = C_IB * o_hat_B * a;
%         positionError = sqrt((desiredPosition - rC_T)'*(desiredPosition - rC_T));

        % The distance:
            r = sqrt(sum(rC_T.^2));

        % Just in case, work out a magnitude for o_hat as well...?
            o_hat = C_IB*o_hat_B;
            o_mag = sqrt(sum(o_hat.^2));
            theta = acos(rC_T'*o_hat/(r*o_mag));
            
        % the dist:
            dist = abs(r-a);
    
    %%%%%%%%%%%%%%%%%%%%%%%%%%%%%%%%%%%%%%%%%%%%%%%%%%%%%%%%%%%
    %%%%%%%%%%% THEN, defining our directions %%%%%%%%%%%%%%%%%
    %%%%%%%%%%%%%%%%%%%%%%%%%%%%%%%%%%%%%%%%%%%%%%%%%%%%%%%%%%%

        
        if theta <= acceptableAngle && dist <= acceptableDistance
            newCnt = currentCnt+1;
        else
            newCnt = 0; % Reset
        end

end

== matlab function tumblingExample/Controlled Spacecraft Dynamics/Gravity ==
  data: R input; R_ddot output; MU parameter
function R_ddot = fcn(R, MU)

r_norm = sqrt(sum(R.^2));
R_ddot = -MU/r_norm^3  *  R;

== matlab function tumblingExample/GNC System/CLVF/Lyapunov Guidance + FF ==
  data: rC_I input; h output; rT_I input; vT_I input; aT_I input; CT_BI input; wT_B input; w_dot_B input; a_ff output; o_hat_B parameter; a parameter; b parameter; ka parameter; kc parameter; vC_I input; r output; newTheta output; o_hat output
function [h, a_ff, r, newTheta, o_hat] = fcn(rC_I, rT_I, vT_I, aT_I, CT_BI, wT_B, w_dot_B, o_hat_B, a, b, ka, kc, vC_I)
    
    % Prep some of the variables for inclusion into the CLVF function:
        C_IB = CT_BI';
        o_hat = C_IB*o_hat_B;
        
%         w_OI = [0;0;theta_dot];
%         w_dot_OI = [0;0;theta_ddot];

        wT_I = C_IB*wT_B;
        w_dot_I = C_IB*w_dot_B;
        
        rC_T = rC_I - rT_I;
        vC_T = vC_I - vT_I;
        
        q = 0.000001; % Small number!
        
        
[h, a_ff, r, newTheta] = CLVF_quad(rC_T, wT_I, w_dot_I, o_hat, vT_I, aT_I, a, b, ka, kc, vC_T, q);

== matlab function tumblingExample/GNC System/PD + FF Controller ==
  data: h input; f output; vC_I input; a_ff input; m parameter; kd parameter
function f = fcn(h, vC_I, a_ff, m, kd)

f = kd*(h - vC_I)+ m*a_ff;
end

== matlab function tumblingExample/Target Dynamics/Target Attitude/Attitude Dynamics ==
  data: w input; w_dot output; I parameter
function w_dot = fcn(w, I)

w_dot = -inv(I)*cross(w,I*w);
